simulink model "net_model_2_nodes"  (R2024a)
settings: Solver=VariableStepAuto  StartTime=0.0  StopTime=n_max  RelTol=1e-3
undefined symbols (not defined in the file): node_1_0, node_2_0, ss_nom
settings Model: Creator=antoniostavarache  LastModifiedBy=antoniostavarache

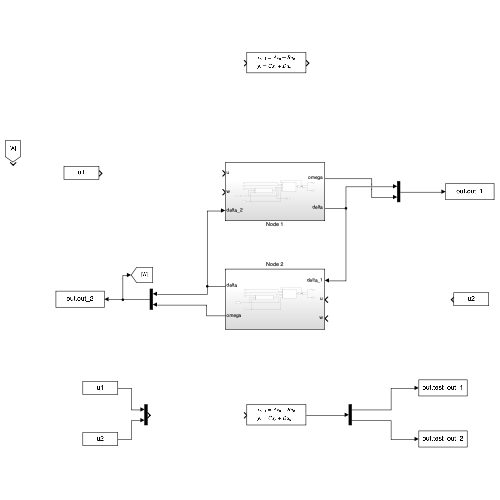
[thumbnail: Simulink's stored preview of the top-level diagram]
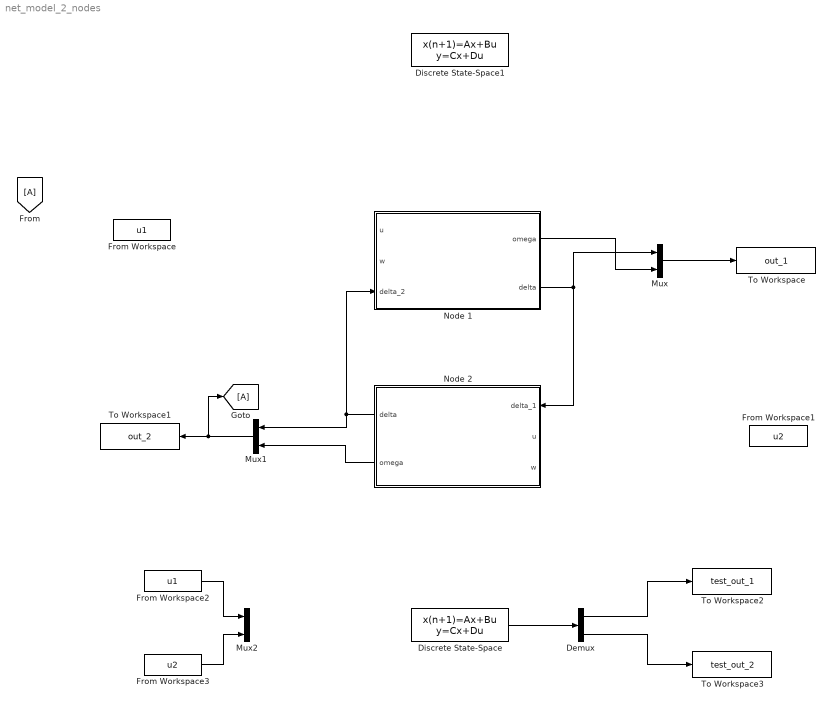
== system net_model_2_nodes ==
  Demux : Demux  Outputs=2
  Discrete State-Space : DiscreteStateSpace  A=ss_nom.A  B=ss_nom.B  C=ss_nom.C  D=ss_nom.D  InitialCondition=[node_1_0; node_2_0]
  Discrete State-Space1 : DiscreteStateSpace  SampleTime=-1
  From : From
  From Workspace : FromWorkspace  VariableName=u1  SampleTime=1
  From Workspace1 : FromWorkspace  VariableName=u2  SampleTime=1
  From Workspace2 : FromWorkspace  VariableName=u1
  From Workspace3 : FromWorkspace  VariableName=u2
  Goto : Goto
  Mux : Mux  Inputs=2
  Mux1 : Mux  Inputs=2
  Mux2 : Mux  Inputs=2
  Node 1 : Subsystem
  Node 2 : Subsystem
  To Workspace : ToWorkspace  VariableName=out_1  SaveFormat=Timeseries  SampleTime=-1
  To Workspace1 : ToWorkspace  VariableName=out_2  SaveFormat=Timeseries  SampleTime=-1
  To Workspace2 : ToWorkspace  VariableName=test_out_1  SaveFormat=Timeseries  SampleTime=-1
  To Workspace3 : ToWorkspace  VariableName=test_out_2  SaveFormat=Timeseries  SampleTime=-1
  wires:
  Node 1/2(delta) -> Node 2/1(delta_1), Mux/1
  Node 2/1(delta) -> Mux1/1, Node 1/3(delta_2)
  Mux/1 -> To Workspace/1
  Mux1/1 -> Goto/1, To Workspace1/1
  Node 2/2(omega) -> Mux1/2
  From Workspace2/1 -> Mux2/1
  From Workspace3/1 -> Mux2/2
  Discrete State-Space/1 -> Demux/1
  Demux/1 -> To Workspace2/1
  Demux/2 -> To Workspace3/1
  Node 1/1(omega) -> Mux/2

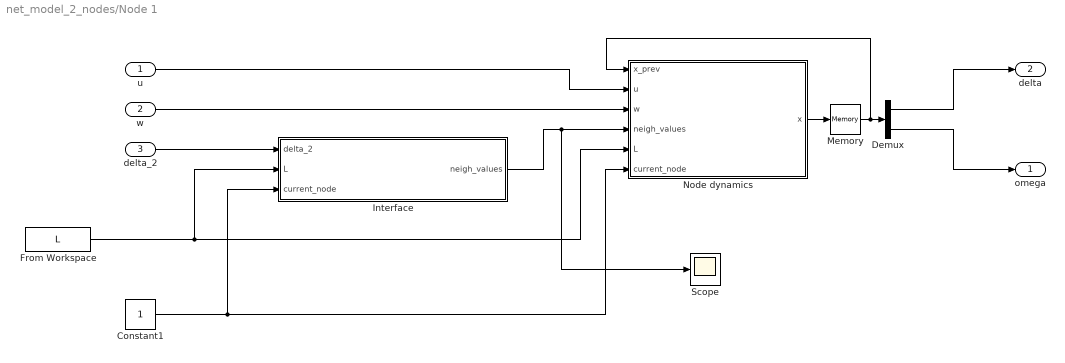
== system net_model_2_nodes/Node 1 ==
  u : Inport
  w : Inport  Port=2
  delta_2 : Inport  Port=3
  Constant1 : Constant
  Demux : Demux  Outputs=2
  From Workspace : FromWorkspace  VariableName=L
  Interface : MATLAB Function  TreatAsAtomicUnit=on
  Memory : Memory  InitialCondition=node_1_0
  Node dynamics : MATLAB Function  TreatAsAtomicUnit=on
  Scope : Scope
  omega : Outport
  delta : Outport  Port=2
  wires:
  Node dynamics/1(x) -> Memory/1
  Interface/1(neigh_values) -> Scope/1, Node dynamics/4(neigh_values)
  From Workspace/1 -> Node dynamics/5(L), Interface/2(L)
  Constant1/1 -> Node dynamics/6(current_node), Interface/3(current_node)
  u/1 -> Node dynamics/2(u)
  w/1 -> Node dynamics/3(w)
  Demux/1 -> delta/1
  Demux/2 -> omega/1
  delta_2/1 -> Interface/1(delta_2)
  Memory/1 -> Node dynamics/1(x_prev), Demux/1

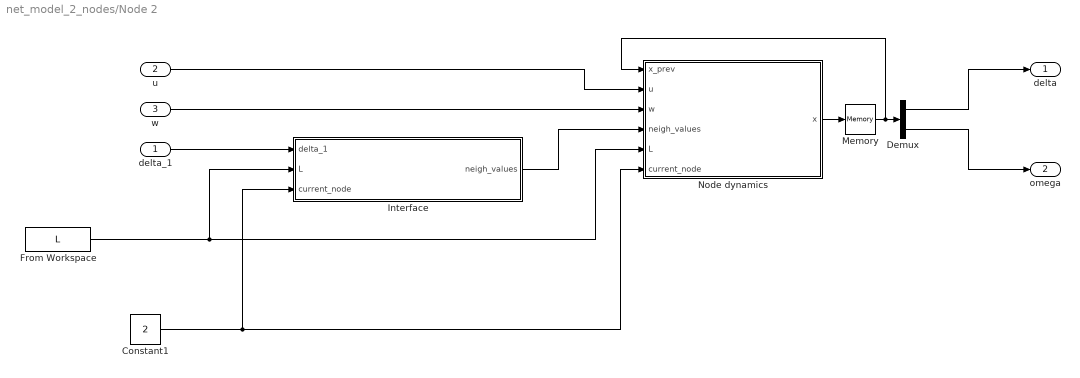
== system net_model_2_nodes/Node 2 ==
  delta_1 : Inport
  u : Inport  Port=2
  w : Inport  Port=3
  Constant1 : Constant  Value=2
  Demux : Demux  Outputs=2
  From Workspace : FromWorkspace  VariableName=L
  Interface : MATLAB Function  TreatAsAtomicUnit=on
  Memory : Memory  InitialCondition=node_2_0
  Node dynamics : MATLAB Function  TreatAsAtomicUnit=on
  delta : Outport
  omega : Outport  Port=2
  wires:
  Node dynamics/1(x) -> Memory/1
  Interface/1(neigh_values) -> Node dynamics/4(neigh_values)
  From Workspace/1 -> Node dynamics/5(L), Interface/2(L)
  Constant1/1 -> Node dynamics/6(current_node), Interface/3(current_node)
  u/1 -> Node dynamics/2(u)
  w/1 -> Node dynamics/3(w)
  Demux/1 -> delta/1
  Demux/2 -> omega/1
  delta_1/1 -> Interface/1(delta_1)
  Memory/1 -> Node dynamics/1(x_prev), Demux/1

== matlab function net_model_2_nodes/Node 1/Interface ==
  data: delta_2 input; neigh_values output; L input; current_node input
function neigh_values = fcn(delta_2, L, current_node)
    
    % curr_node = 1;

    % l_mat = [0 0.6511 0.7915 0 0.7513;
    %     0.6511 0 0 0.8433 0.6318;
    %     0.7915 0 0 0.8259 0.8620;
    %     0 0.8433 0.8259 0 0.8367;
    %     0.7513 0.6318 0.8620 0.8367 0];

    l_mat = [0 0.6511;
        0.6511 0];

    neigh_values = L(current_node, 2) * l_mat(current_node, 2) * delta_2;

end

== matlab function net_model_2_nodes/Node 1/Node dynamics ==
  data: x_prev input; u input; x output; w input; neigh_values input; L input; current_node input
function x = fcn(x_prev, u, w, neigh_values, L, current_node)
    
    % current_node = 1;

%%

    hi = [0.3244
        1.5886];

    di = [0.5650;
        0.7844];
    
    l_mat = [0 0.6511;
        0.6511 0];

    dt = 0.2;
%%

    a21 = -hi(current_node) * dt * L(current_node, :) * l_mat(current_node, :)';
    a22 = 1 - hi(current_node) * di(current_node) * dt;

    A = [1, dt;
        a21, a22];

    x = A * x_prev + [0 1]' * (u + w + hi(current_node) * dt * neigh_values);
    
end

== matlab function net_model_2_nodes/Node 2/Interface ==
  data: delta_1 input; neigh_values output; L input; current_node input
function neigh_values = fcn(delta_1, L, current_node)
    
    % curr_node = 1;

    % l_mat = [0 0.6511 0.7915 0 0.7513;
    %     0.6511 0 0 0.8433 0.6318;
    %     0.7915 0 0 0.8259 0.8620;
    %     0 0.8433 0.8259 0 0.8367;
    %     0.7513 0.6318 0.8620 0.8367 0];

    l_mat = [0 0.6511;
        0.6511 0];

    neigh_values = L(current_node, 1) * l_mat(current_node, 1) * delta_1;

end

== matlab function net_model_2_nodes/Node 2/Node dynamics ==
  data: x_prev input; u input; x output; w input; neigh_values input; L input; current_node input
function x = fcn(x_prev, u, w, neigh_values, L, current_node)
    
    % current_node = 1;

%%

    hi = [0.3244
        1.5886];

    di = [0.5650;
        0.7844];
    
    l_mat = [0 0.6511;
        0.6511 0];

    dt = 0.2;
    
%%

    a21 = -hi(current_node) * dt * L(current_node, :) * l_mat(current_node, :)';
    a22 = 1 - hi(current_node) * di(current_node) * dt;

    A = [1, dt;
        a21, a22];

    x = A * x_prev + [0 1]' * (u + w + hi(current_node) * dt * neigh_values);
    
end
